simulink model "system_model_linearization_v2_2021"  (R2022b)
settings: Solver=ode4  StartTime=0.0  StopTime=10  RelTol=1e-3
values from neighbouring files (symbols this model uses):
  A = [0 1 0 0 ... (first row only)    [linearize_script.m]    (also in step4_0_linearize_operating_point.m = double(A); step4_linearized_system.mat = [0 0.306815158551 0 -109.913929424 0 1 -60.0152130057 0 126.; syms_test.m = double(A))
  B = [0 ... (first row only)    [linearize_script.m]    (also in step4_0_linearize_operating_point.m = double(B); step4_linearized_system.mat = [0 0 0 0 858.38566108]; syms_test.m = double(B))
  C = [1 0 0 0 ... (first row only)    [linearize_script.m]    (also in matrixmaker_linearization.m = [b_1_0 - P_3 * theta_d_2 * sin(theta_2)  -P_3 * (theta_d_1 +; step4_0_linearize_operating_point.m = [1 0 0 0 0; step4_linearized_system.mat = [1  0  0  0  0; 0  0  1  0  0]; syms_test.m)
  D = zeros(2,1)    [linearize_script.m]    (also in step4_0_linearize_operating_point.m; step4_linearized_system.mat = [0 0]; syms_test.m)
  init_theta_1 = pi    (= 3.14159265359)    [Copy_of_step2_whitebox_beam.m]    (also in compare_ourmodel_with_others.m = 0; linearize_script.m; step2_whitebox_beam.m; syms_test.m)
  init_theta_2 = -pi/2    (= -1.57079632679)    [Copy_of_step2_whitebox_beam.m]    (also in compare_ourmodel_with_others.m = 0; linearize_script.m = 1.57079632679; step2_whitebox_beam.m; syms_test.m = 0)
  x0 = [pi; 0]    [linearization.m]    (also in linearize_script.m = [init_theta_1;0;init_theta_2;0]; linearize_test_script.m = [pi 0]; syms_test.m = [init_theta_1; 0; init_theta_2; 0])
settings Model: Creator=97083  LastModifiedBy=annel
settings DataIOCC: ExternalInput=[u]
settings DebuggingCC: UnderSpecifiedDimensionMsg=warning

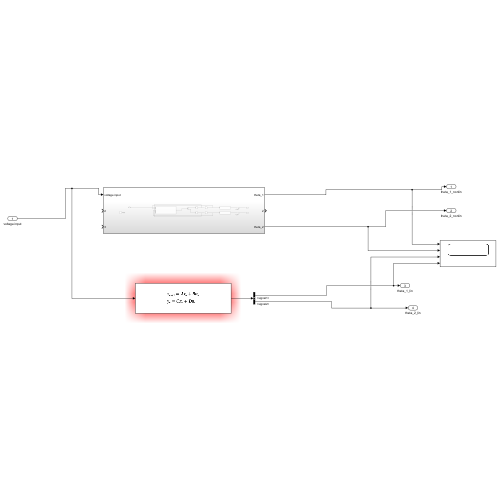
[thumbnail: Simulink's stored preview of the top-level diagram]
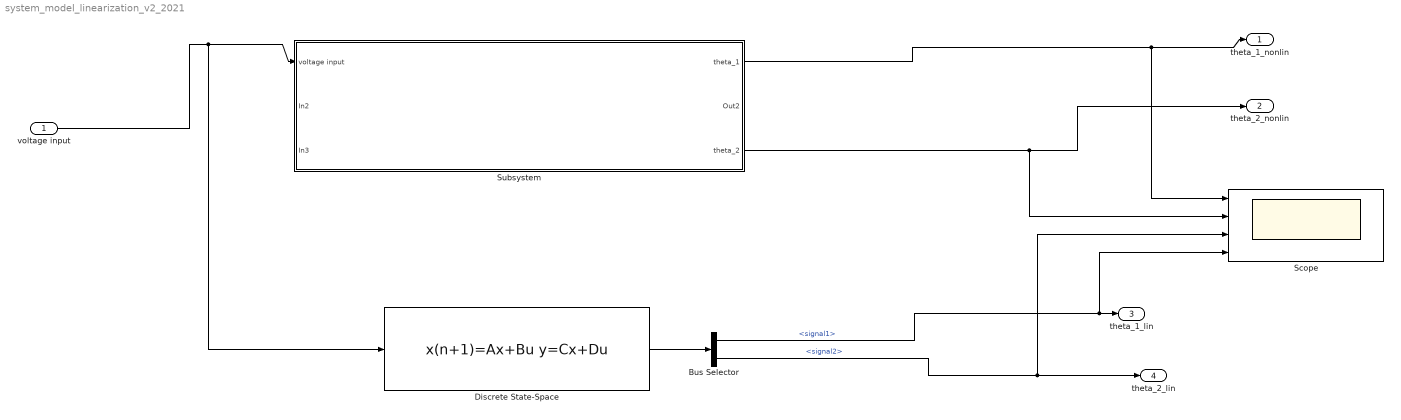
== system system_model_linearization_v2_2021 ==
  voltage input : Inport  PortDimensions=1  LockScale=on
  Bus Selector : BusSelector  OutputSignals=signal1,signal2
  Discrete State-Space : DiscreteStateSpace  A=A  B=B  C=C  D=D  InitialCondition=x0  SampleTime=-1
  Scope : Scope  NumInputPorts=4
  Subsystem : Subsystem
  theta_1_nonlin : Outport
  theta_2_nonlin : Outport  Port=2
  theta_1_lin : Outport  Port=3
  theta_2_lin : Outport  Port=4
  wires:
  voltage input/1 -> Discrete State-Space/1, Subsystem/1(voltage input)
  Subsystem/1(theta_1) -> Scope/1, theta_1_nonlin/1
  Subsystem/3(theta_2) -> Scope/2, theta_2_nonlin/1
  Discrete State-Space/1 -> Bus Selector/1
  Bus Selector/1 -> Scope/4, theta_1_lin/1  "<signal1>"
  Bus Selector/2 -> Scope/3, theta_2_lin/1  "<signal2>"

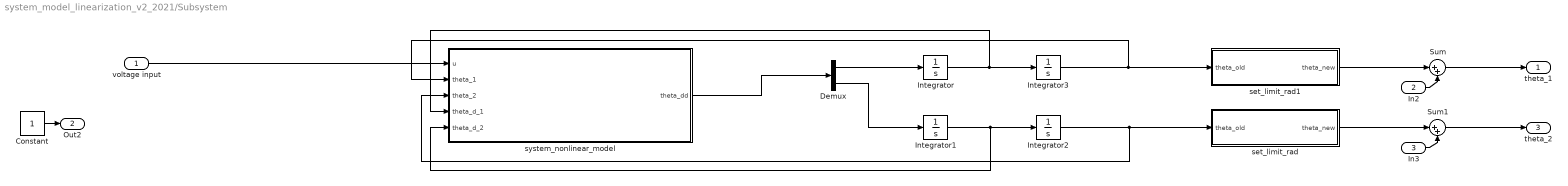
== system system_model_linearization_v2_2021/Subsystem ==
  voltage input : Inport  PortDimensions=1  LockScale=on
  In2 : Inport  Port=2
  In3 : Inport  Port=3
  Constant : Constant
  Demux : Demux  Outputs=2
  Integrator : Integrator
  Integrator1 : Integrator
  Integrator2 : Integrator  InitialCondition=init_theta_2
  Integrator3 : Integrator  InitialCondition=init_theta_1
  Sum : Sum  Inputs=|++
  Sum1 : Sum  Inputs=|++
  set_limit_rad : MATLAB Function  TreatAsAtomicUnit=on
  set_limit_rad1 : MATLAB Function  TreatAsAtomicUnit=on
  system_nonlinear_model : MATLAB Function  TreatAsAtomicUnit=on
  theta_1 : Outport
  Out2 : Outport  Port=2
  theta_2 : Outport  Port=3
  wires:
  Demux/1 -> Integrator/1
  Sum1/1 -> theta_2/1
  Integrator2/1 -> system_nonlinear_model/3(theta_2), set_limit_rad/1(theta_old)
  Integrator/1 -> system_nonlinear_model/4(theta_d_1), Integrator3/1
  Integrator3/1 -> set_limit_rad1/1(theta_old), system_nonlinear_model/2(theta_1)
  In3/1 -> Sum1/2
  Integrator1/1 -> system_nonlinear_model/5(theta_d_2), Integrator2/1
  system_nonlinear_model/1(theta_dd) -> Demux/1
  set_limit_rad1/1(theta_new) -> Sum/1
  set_limit_rad/1(theta_new) -> Sum1/1
  voltage input/1 -> system_nonlinear_model/1(u)
  Demux/2 -> Integrator1/1
  Sum/1 -> theta_1/1
  In2/1 -> Sum/2
  Constant/1 -> Out2/1

== matlab function system_model_linearization_v2_2021/Subsystem/set_limit_rad ==
  settings: updateMethod=DISCRETE  sampleTime=0.001
  data: theta_old input size=1; theta_new output size=1
function theta_new   = set_limit_rad(theta_old)

theta_new = theta_old - floor(theta_old / 2 / pi) * 2 * pi;
theta_new = theta_old;

== matlab function system_model_linearization_v2_2021/Subsystem/system_nonlinear_model ==
  settings: updateMethod=DISCRETE  sampleTime=0.001
  data: u input size=1; theta_dd output size=2; theta_1 input size=1; theta_2 input size=1; theta_d_1 input size=1; theta_d_2 input size=1
function theta_dd   = get_theta_dt_dt(u, theta_1, theta_2, theta_d_1, theta_d_2)

% constant variables
g = 9.81;
l_1 = 0.1;
l_2 = 0.1;
m_1 = 0.125;
m_2 = 0.05;
params = [-0.001, 0.077, 0.2, 0.00004, 20.684, 0.0004, 15, 0.03];
% params = [-0.04, 0.06, 0.074, 0.00002, 4.8, 0.00077, 50, 0.03];

% varying variables
c_1_0 = params(1);
c_2_0 = params(2);
I_1_0 = params(3);
I_2_0 = params(4);
b_1_0 = params(5);
b_2_0 = params(6);
k_m_0 = params(7);
tau_e_0 = params(8);


% calculate other variables
P_1 = m_1 * c_1_0 * c_1_0 + m_2 * l_1 * l_1 + I_1_0;
P_2 = m_2 * c_2_0 * c_2_0 + I_2_0;
P_3 = m_2 * l_1 * c_2_0;

g_1 = (m_1 * c_1_0 + m_2 * l_1) * g;
g_2 = m_2 * c_2_0 * g;


% construct the vector for matrix calculation

% theta_vec = [theta_1; theta_2];
theta_d_vec = [theta_d_1; theta_d_2];
% theta_d_d_vec = [theta_1; theta_2];
T = k_m_0 * u;
T_vec = [T; 0];
theta_dd = zeros(2, 1);

% matrix
M = [P_1 + P_2 + 2 * P_3 * cos(theta_2) P_2 + P_3 * cos(theta_2);
    P_2 + P_3 * cos(theta_2)            P_2];

C = [b_1_0 - P_3 * theta_d_2 * sin(theta_2)  -P_3 * (theta_d_1 + theta_d_2) * sin(theta_2);
    P_3 * theta_d_1 * sin(theta_2)           b_2_0];

G = [-g_1 * sin(theta_1) - g_2 * sin(theta_1 + theta_2);
     -g_2 * sin(theta_1 + theta_2)];

M_inv = inv(M);

theta_dd = M_inv * T_vec - M_inv * C * theta_d_vec- M_inv * G;

== matlab function system_model_linearization_v2_2021/Subsystem/set_limit_rad1 ==
  settings: updateMethod=DISCRETE  sampleTime=0.001
  data: theta_old input size=1; theta_new output size=1
function theta_new   = set_limit_rad(theta_old)

theta_new = theta_old - floor(theta_old / 1.5 / pi) * 2 * pi;
theta_new = theta_old;
